simulink model "ball_table_with_pid"  (R2015a)
settings: Solver=ode45  StartTime=0.0  StopTime=10.0  RelTol=1e-3
undefined symbols (not defined in the file or in its folder): B, g, M
libraries: vrlib x4, simulink x2
settings Model: Creator=PC  LastModifiedBy=PC

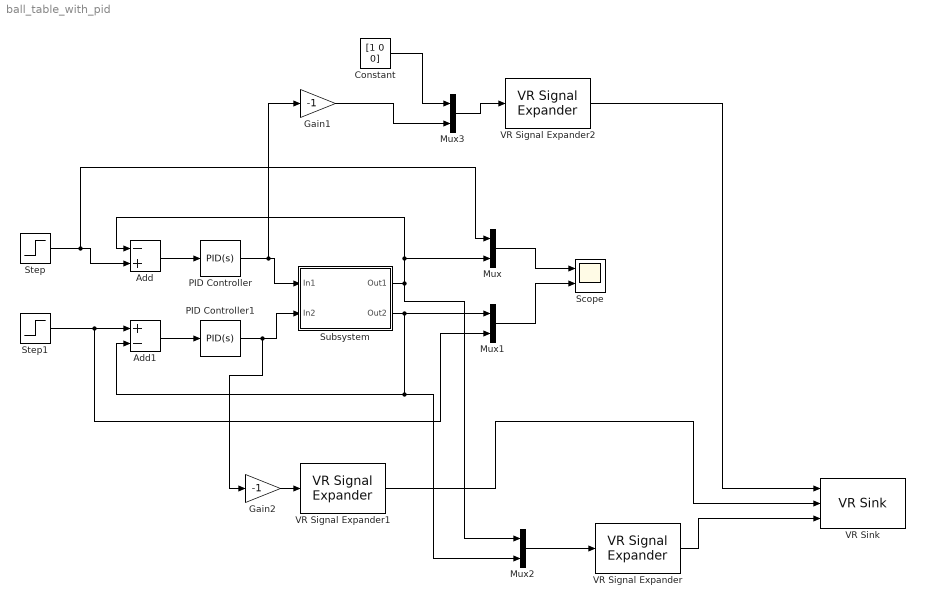
== system ball_table_with_pid ==
  Add : Sum  Inputs=-+
  Add1 : Sum  Inputs=+-
  Constant : Constant  Value=[1 0 0]
  Gain1 : Gain  Gain=-1
  Gain2 : Gain  Gain=-1
  Mux{,1..3} (4 alike) : Mux  Inputs=2
  PID Controller : simulink/Continuous/PID Controller  Controller=PID  TimeDomain=Continuous-time  SampleTime=-1  IntegratorMethod=Forward Euler  FilterMethod=Forward Euler  Form=Parallel  UseFilter=on  ControllerParametersSource=internal  P=1  I=0  D=1  N=100  InitialConditionSource=internal  InitialConditionForIntegrator=0  InitialConditionForFilter=0  ExternalReset=none  LimitOutput=off  UpperSaturationLimit=inf  LowerSaturationLimit=-inf  LinearizeAsGain=on  AntiWindupMode=none  Kb=1  TrackingMode=off  Kt=1  PParamMin=[]  PParamMax=[]  IParamMin=[]  IParamMax=[]  DParamMin=[]  DParamMax=[]  NParamMin=[]  NParamMax=[]  KbParamMin=[]  KbParamMax=[]  KtParamMin=[]  KtParamMax=[]  POutMin=[]  POutMax=[]  IOutMin=[]  IOutMax=[]  DOutMin=[]  DOutMax=[]  NOutMin=[]  NOutMax=[]  KbOutMin=[]  KbOutMax=[]  KtOutMin=[]  KtOutMax=[]  IntegratorOutMin=[]  IntegratorOutMax=[]  FilterOutMin=[]  FilterOutMax=[]  SumOutMin=[]  SumOutMax=[]  SumI1OutMin=[]  SumI1OutMax=[]  SumI2OutMin=[]  SumI2OutMax=[]  SumI3OutMin=[]  SumI3OutMax=[]  SumDOutMin=[]  SumDOutMax=[]  SaturationOutMin=[]  SaturationOutMax=[]  IntegratorContinuousStateAttributes=''  IntegratorStateMustResolveToSignalObject=off  IntegratorRTWStateStorageClass=Auto  FilterContinuousStateAttributes=''  FilterStateMustResolveToSignalObject=off  FilterRTWStateStorageClass=Auto  DifferentiatorICPrevScaledInput=0  DifferentiatorOutMin=[]  DifferentiatorOutMax=[]
  PID Controller1 : simulink/Continuous/PID Controller  Controller=PID  TimeDomain=Continuous-time  SampleTime=-1  IntegratorMethod=Forward Euler  FilterMethod=Forward Euler  Form=Parallel  UseFilter=on  ControllerParametersSource=internal  P=1  I=0  D=1  N=100  InitialConditionSource=internal  InitialConditionForIntegrator=0  InitialConditionForFilter=0  ExternalReset=none  LimitOutput=off  UpperSaturationLimit=inf  LowerSaturationLimit=-inf  LinearizeAsGain=on  AntiWindupMode=none  Kb=1  TrackingMode=off  Kt=1  PParamMin=[]  PParamMax=[]  IParamMin=[]  IParamMax=[]  DParamMin=[]  DParamMax=[]  NParamMin=[]  NParamMax=[]  KbParamMin=[]  KbParamMax=[]  KtParamMin=[]  KtParamMax=[]  POutMin=[]  POutMax=[]  IOutMin=[]  IOutMax=[]  DOutMin=[]  DOutMax=[]  NOutMin=[]  NOutMax=[]  KbOutMin=[]  KbOutMax=[]  KtOutMin=[]  KtOutMax=[]  IntegratorOutMin=[]  IntegratorOutMax=[]  FilterOutMin=[]  FilterOutMax=[]  SumOutMin=[]  SumOutMax=[]  SumI1OutMin=[]  SumI1OutMax=[]  SumI2OutMin=[]  SumI2OutMax=[]  SumI3OutMin=[]  SumI3OutMax=[]  SumDOutMin=[]  SumDOutMax=[]  SaturationOutMin=[]  SaturationOutMax=[]  IntegratorContinuousStateAttributes=''  IntegratorStateMustResolveToSignalObject=off  IntegratorRTWStateStorageClass=Auto  FilterContinuousStateAttributes=''  FilterStateMustResolveToSignalObject=off  FilterRTWStateStorageClass=Auto  DifferentiatorICPrevScaledInput=0  DifferentiatorOutMin=[]  DifferentiatorOutMax=[]
  Scope : Scope  NumInputPorts=2
      settings: YMin=-5~-5  YMax=5~5
  Step : Step  Time=5  SampleTime=0
  Step1 : Step  SampleTime=0
  Subsystem : Subsystem
  VR Signal Expander : vrlib/VR Signal Expander  outwidth=3  outidx=[1 3]
  VR Signal Expander1 : vrlib/VR Signal Expander  outwidth=4  outidx=[4]
  VR Signal Expander2 : vrlib/VR Signal Expander  outwidth=4  outidx=[1 2 3 4]
  VR Sink : vrlib/VR Sink  InstantiateOnLoad=on  SampleTime=0.1  ViewEnable=on  RemoteChange=off  RemoteView=off  FieldsWritten=Tablex.rotation.4.1.1.double#Table_y.rotation.4.1.1.double#Ball.translation.3.1.1.double  WorldFileName=model3D.wrl  AutoView=off  VideoDimensions=[]  AllowVariableSize=off
  wires:
  Add/1 -> PID Controller/1
  PID Controller/1 -> Gain1/1, Subsystem/1(In1)
  PID Controller1/1 -> Gain2/1, Subsystem/2(In2)
  Add1/1 -> PID Controller1/1
  Step1/1 -> Mux1/2, Add1/1
  Subsystem/1(Out1) -> Mux/2, Add/1, Mux2/1
  Subsystem/2(Out2) -> Mux1/1, Mux2/2, Add1/2
  Mux1/1 -> Scope/2
  Mux/1 -> Scope/1
  Mux2/1 -> VR Signal Expander/1
  VR Signal Expander/1 -> VR Sink/3
  VR Signal Expander1/1 -> VR Sink/2
  Step/1 -> Mux/1, Add/2
  VR Signal Expander2/1 -> VR Sink/1
  Gain2/1 -> VR Signal Expander1/1
  Gain1/1 -> Mux3/2
  Constant/1 -> Mux3/1
  Mux3/1 -> VR Signal Expander2/1

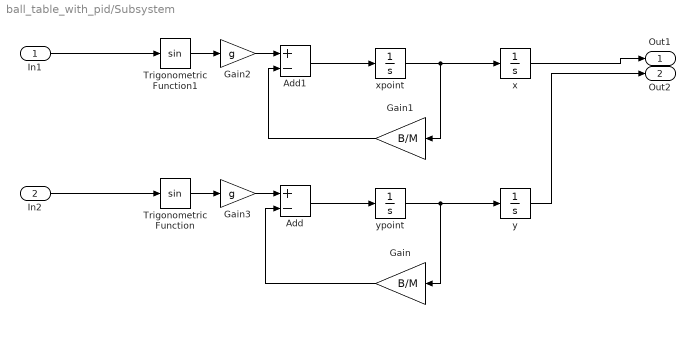
== system ball_table_with_pid/Subsystem ==
  In1 : Inport
  In2 : Inport  Port=2
  Add : Sum  Inputs=+-
  Add1 : Sum  Inputs=+-
  Gain : Gain  Gain=B/M
  Gain1 : Gain  Gain=B/M
  Gain2 : Gain  Gain=g
  Gain3 : Gain  Gain=g
  Trigonometric Function : Trigonometry
  Trigonometric Function1 : Trigonometry
  x : Integrator
  xpoint : Integrator
  y : Integrator
  ypoint : Integrator
  Out1 : Outport
  Out2 : Outport  Port=2
  wires:
  Gain2/1 -> Add1/1
  Trigonometric Function1/1 -> Gain2/1
  Gain3/1 -> Add/1
  Trigonometric Function/1 -> Gain3/1
  Gain/1 -> Add/2
  Gain1/1 -> Add1/2
  Add1/1 -> xpoint/1
  Add/1 -> ypoint/1
  In2/1 -> Trigonometric Function/1
  In1/1 -> Trigonometric Function1/1
  ypoint/1 -> y/1, Gain/1
  xpoint/1 -> x/1, Gain1/1
  x/1 -> Out1/1
  y/1 -> Out2/1
